simulink model "fig7_45"  (Simulink 4.00)
settings: Solver=ode45  StartTime=0.0  StopTime=100.0  RelTol=1e-3
undefined symbols (not defined in the file or in its folder): aa, bb, cc, dd
libraries: simulink3 x1
settings Model: LastModifiedBy=abbas  LimitDataPoints=off  ExtModeTrigMode=oneshot  ExtModeArmWhenConnect=off  BlockReductionOpt=off

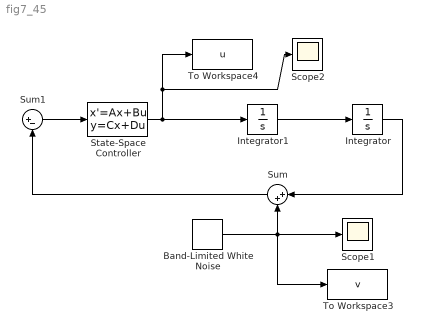
== system fig7_45 ==
  Band-Limited White Noise : simulink3/Sources/Band-Limited White Noise  Cov=[0.1]  Ts=0.05  seed=[23341]
  Integrator : Integrator  ExternalReset=none  InitialConditionSource=internal  InitialCondition=0  LimitOutput=off  UpperSaturationLimit=inf  LowerSaturationLimit=-inf  ShowSaturationPort=off  ShowStatePort=off  AbsoluteTolerance=auto
  Integrator1 : Integrator  ExternalReset=none  InitialConditionSource=internal  InitialCondition=0  LimitOutput=off  UpperSaturationLimit=inf  LowerSaturationLimit=-inf  ShowSaturationPort=off  ShowStatePort=off  AbsoluteTolerance=auto
  Scope1 : Scope
      settings: TimeRange=auto  YMin=-12.5  YMax=10  SaveToWorkspace=off  SaveName=ScopeData  LimitDataPoints=on  MaxDataPoints=5000
  Scope2 : Scope
      settings: TimeRange=auto  YMin=-12.5  YMax=10  SaveToWorkspace=off  SaveName=ScopeData  LimitDataPoints=on  MaxDataPoints=5000
  State-Space Controller : StateSpace  A=aa  B=bb  C=cc  D=dd  X0=0  Realization=auto  AbsoluteTolerance=auto
  Sum : Sum  Orientation=left  Inputs=|++  SaturateOnIntegerOverflow=on
  Sum1 : Sum  Inputs=|+-  SaturateOnIntegerOverflow=on
  To Workspace3 : ToWorkspace  VariableName=v  SampleTime=0.0  SaveFormat=Array
  To Workspace4 : ToWorkspace  VariableName=u  SampleTime=0.0  SaveFormat=Array
  wires:
  Integrator1/1 -> Integrator/1
  Integrator/1 -> Sum/1
  Sum/1 -> Sum1/2
  Sum1/1 -> State-Space Controller/1
  Band-Limited White Noise/1 -> Sum/2, Scope1/1, To Workspace3/1
  State-Space Controller/1 -> Integrator1/1, To Workspace4/1, Scope2/1
